simulink model "WaterRunner_closed"  (Simulink 8.0)
settings: Solver=ode15s  StartTime=0.0  StopTime=10  FixedStep=1e-3  RelTol=1e-3
values from neighbouring files (symbols this model uses):
  Amp = leg_length    (= 0.0428)    [SimParam.m]    (also in simParams_closed.m = 0.0249)
  b_water = 0.5*C_d*S1*density    (= 0.405708731037)    [SimParam.m]    (also in simParams_closed.m)
  D = 2*pi    (= 6.28318530718)    [DF_param.m]
  Filter_Coef = 1000    [SimParam.m]    (also in simParams_closed.m)
  frame_inertia = diag([Ix,Iy,Iz])    [SimParam.m]    (also in matlab.mat = [8.0125e-05  0  0; 0  0.000390625  0; 0  0  0.0003145]; simParams.m; simParams_closed.m; speed_cg.mat = [8.0125e-05  0  0; 0  0.000390625  0; 0  0  0.0003145])
  frame_mass = 0.06    [matlab.mat]    (also in simParam.m = 0.03; simParams.m; simParams_closed.m = 0.1; speed_cg.mat)
  Fratio = 1/16    (= 0.0625)    [SimParam.m]    (also in simParams_closed.m)
  g = 9.81    [SimParam.m]    (also in linear_search_df.m; simParams_closed.m)
  k_water = C_d*S1*density*g    (= 7.96000530294)    [SimParam.m]    (also in simParams_closed.m)
  L2_inertia = [1.05087286587e-08  0  0; 0  0  0; 0  0  1.05087286587e-08]    [matlab.mat]    (also in simParams.m = diag([I 0 I]); simParams_closed.m = diag([I 0 I]); speed_cg.mat)
  L2_mass = 0.0002653496    [matlab.mat]    (also in simParams.m; simParams_closed.m; speed_cg.mat)
  L3_inertia = [4.24507620885e-07  0  0; 0  0  0; 0  0  4.24507620885e-07]    [matlab.mat]    (also in simParams.m = diag([I 0 I]); simParams_closed.m = diag([I 0 I]); speed_cg.mat)
  L3_mass = 0.0009104656    [matlab.mat]    (also in simParams.m; simParams_closed.m; speed_cg.mat)
  L4_inertia = [1.03972444992e-07  0  0; 0  0  0; 0  0  1.03972444992e-07]    [matlab.mat]    (also in simParams.m = diag([I 0 I]); simParams_closed.m = diag([I 0 I]); speed_cg.mat)
  L4_mass = 0.0005696496    [matlab.mat]    (also in simParams.m; simParams_closed.m; speed_cg.mat)
  leg_length = 0.0428    [SimParam.m]    (also in simParams_closed.m = 0.0249)
  Lx = frame_width/2*[1 1 -1 -1]'    [SimParam.m]    (also in simParams_closed.m)
  Lxmat = frame_width/2*[1 0 0 0 ; 0 1 0 0 ; 0 0 -1 0 ; 0 0 0 -1]    [SimParam.m]    (also in simParams_closed.m)
  Lz = frame_length/2*[1 -1 -1 1]'    [SimParam.m]    (also in simParams_closed.m)
  Lzmat = frame_length/2*[1 0 0 0 ; 0 -1 0 0 ; 0 0 -1 0 ; 0 0 0 1]    [SimParam.m]    (also in simParams_closed.m)
  mass = 0.1    [SimParam.m]    (also in simParams_closed.m = 0.1581990592)
  mass_matrix = [mass 0 0; 0 Ix 0 ; 0 0 Iz]    [SimParam.m]    (also in simParams_closed.m)
  omega_0 = freq*ones(8,1)    [SimParam.m]    (also in simParams_closed.m)
  water_level = 0    [matlab.mat]    (also in simParam.m; simParams.m; simParams_closed.m; speed_cg.mat)
undefined symbols (not defined in the file): cw_FL_HL, cw_FR_FL, cw_FR_HR, cw_HR_HL, FL_HL_lag, FR_FL_lag, FR_HR_lag, freq, HR_HL_lag, initRobHeight, K_d, K_i, K_p, y_0
libraries: mblibv1 x17, WaterRunner_lib x14, dspstat3 x4, simulink x1, dspinverses x1
settings Model: Creator=fumiyaiida  LastModifiedBy=nitisht  SimulationMode=accelerator
settings SolverCC: ZeroCrossControl=DisableAll
settings DataIOCC: SignalLoggingSaveFormat=ModelDataLogs
settings OptimizationCC: InlineInvariantSignals=on  InitFltsAndDblsToZero=on  EfficientMapNaN2IntZero=off  SimCompilerOptimization=On
settings DebuggingCC: SaveWithParameterizedLinksMsg=none  SignalResolutionControl=TryResolveAllWithWarning  SolverPrmCheckMsg=none  MultiTaskDSMMsg=warning  MultiTaskCondExecSysMsg=none  FcnCallInpInsideContextMsg=UseLocalSettings  StrictBusMsg=None
settings HardwareCC: ProdBitPerLong=64  ProdBitPerPointer=64  ProdIntDivRoundTo=Zero  ProdEndianess=LittleEndian  ProdWordSize=64  ProdHWDeviceType=Intel->x86-64  TargetBitPerLong=64  TargetBitPerPointer=64  TargetIntDivRoundTo=Zero  TargetEndianess=LittleEndian  TargetWordSize=64  TargetHWDeviceType=MATLAB Host  ProdEqTarget=off
settings RTWCC: RTWCompilerOptimization=On
settings CodeAppCC: MaxIdLength=128
settings GRTTargetCC: CombineOutputUpdateFcns=off  GRTInterface=on
settings SimMechanicsCC: WarnOnSingularInitialAssembly=on  VisDuringSimulation=on  VisSampleTime=0.001  AnimationDelay=1  LastVizWinPosition=[1323 2 597 976]  CamPosition=[-7.43826;3.54067;9.27536;]  CamTarget=[0.848137;-0.562095;-0.541519;]  CamUpVector=[0.217493;0.952228;-0.21438;]  CamHeight=2.55  VisBackgroundColor=[0.9;0.9;0.95;]  DefaultBodyColor=[1;0;0;]
settings ConfigurationSet: Description=SimMechanics 2G

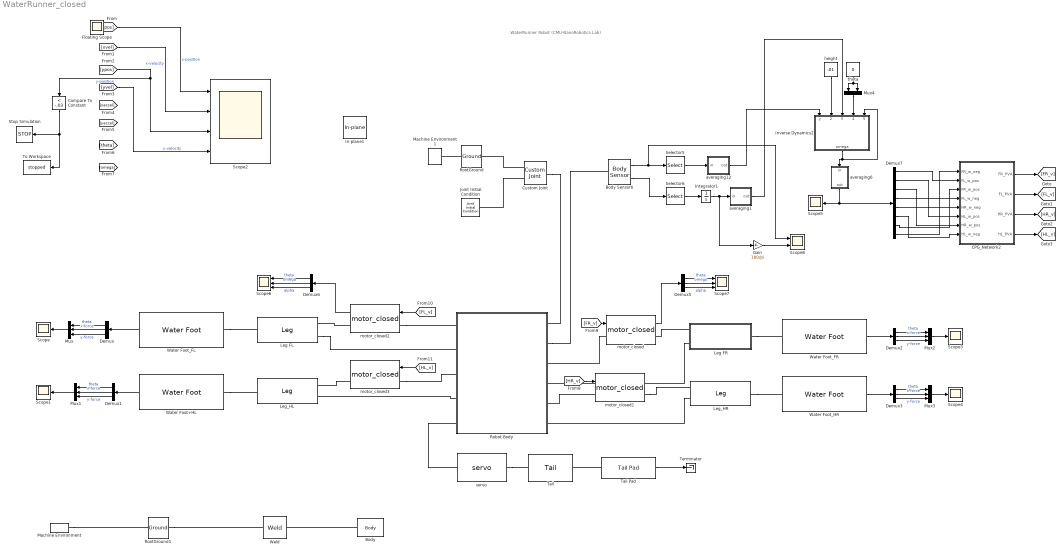
== system WaterRunner_closed ==
  note: WaterRunner Robot
      | (CMU-NanoRobotics Lab)
  Body : mblibv1/Bodies/Body  LConnTagsString=CG  UpdateFromCAD=off  DialogClass=MechanicalBodyBlock  Mass=1  MassUnits=kg  InertiaUnits=kg*m^2  Inertia=eye(3)  Shape=Cylinder  ShapeDims=[1 1]  ShapeUnits=m  ShapeUse=false  Density=1  DensityUnits=kg/m^3  DensityUse=false  GraphicsMode=CONVHULL  BodyColorSelMode=COLORPALETTE  BodyColor=[0.83137 0.81569 0.78431]  AttachedToCS=CG  CG=Left$CG$[0 0 0]$WORLD$WORLD$m$[0 0 0]$Euler X-Y-Z$deg$WORLD$true$none  WorkingFrames=Left$CS1$[-0.5 water_level -0.2 ]$CG$CG$m$[0 0 0]$Euler X-Y-Z$deg$WORLD$false$none#Left$CS2$[-0.5 water_level 0.2 ]$CG$CG$m$[0 0 0]$Euler X-Y-Z$deg$WORLD$false$none#Left$CS3$[4 water_level -0.2 ]$CG$CG$m$[0 0 0]$Euler X-Y-Z$deg$WORLD$false$none#Left$CS4$[4 water_level 0.2 ]$CG$CG$m$[0 0 0]$Euler X-Y-Z$deg$WORLD$false$none  CGPos=[0 0 0]  CGRot=[0 0 0]  CS0Pos=[]  CS0Rot=[]  CS1Pos=[-0.5 water_level -0.2 ]  CS1Rot=[0 0 0]  CS2Pos=[-0.5 water_level 0.2 ]  CS2Rot=[0 0 0]  CS3Pos=[4 water_level -0.2 ]  CS3Rot=[0 0 0]  CS4Pos=[4 water_level 0.2 ]  CS4Rot=[0 0 0]  CS5Pos=[]  CS5Rot=[]  CS6Pos=[]  CS6Rot=[]  CS7Pos=[]  CS7Rot=[]  CS8Pos=[]  CS8Rot=[]  CS9Pos=[]  CS9Rot=[]  CS10Pos=[]  CS10Rot=[]  CS11Pos=[]  CS11Rot=[]  CS12Pos=[]  CS12Rot=[]  CS13Pos=[]  CS13Rot=[]  CS14Pos=[]  CS14Rot=[]  CS15Pos=[]  CS15Rot=[]  CS16Pos=[]  CS16Rot=[]  CS17Pos=[]  CS17Rot=[]  CS18Pos=[]  CS18Rot=[]  CS19Pos=[]  CS19Rot=[]  CS20Pos=[]  CS20Rot=[]
  Body Sensor6 : mblibv1/Sensors &  Actuators/Body Sensor  UpdateFromCAD=off  PhysicalDomain=Mechanical  PortType=blob  Muxed=off  Pose=off  Angle=on  AngleUnits=deg  ArcVelocity=on  ArcVelocityUnits=rad/s  ArcAcceleration=off  ArcAccelerationUnits=deg/s^2  CoordPosition=on  CoordPositionUnits=m  Velocity=off  VelocityUnits=m/s  Acceleration=off  AccelerationUnits=m/s^2  Quaternion=on  QuaternionDT=off  QuaternionDDT=off  QuaternionUnits=off  OutputVector=[1]  ActiveIO=on  Width=6  DialogClass=MechanicalSensorBlock  ReferenceFrame=Absolute (World)
  CPG_Network2 : Subsystem
  Compare To Constant : simulink/Logic and Bit Operations/Compare To Constant  relop=<  const=-.03  OutDataTypeStr=boolean
  Custom Joint : mblibv1/Joints/Custom Joint  LConnTagsString=__newl0|SA1  RConnTagsString=__newr0  UpdateFromCAD=off  NumSAPorts=1  CutJoint=off  MarkAsCut=off  Primitives=prismatic  PrimitiveProps=P1$World$[0 1 0]$Prismatic#P2$World$[1 0 0]$Prismatic#R1$World$[1 0 0]$Revolute#R2$World$[0 0 1]$Revolute  DialogClass=JointBlock  R1Axis=[1 0 0]  R2Axis=[0 0 1]  R3Axis=[]  P1Axis=[0 1 0]  P2Axis=[1 0 0]  P3Axis=[]  SAxis=[]
  Demux{,1..3,5..6} (6 alike) : Demux  Outputs=3
  Demux7 : Demux  Outputs=8
  Gain : Gain  Gain=180/pi
  In-plane1 : mblibv1/Joints/In-plane  LConnTagsString=__newl0|SA1|SA2  RConnTagsString=__newr0|SA1|SA2  UpdateFromCAD=off  NumSAPorts=4  CutJoint=off  MarkAsCut=off  Primitives=prismatic  PrimitiveProps=P1$World$[1 0 0]$prismatic#P2$World$[0 1 0]$prismatic  DialogClass=JointBlock  P1Axis=[1 0 0]  P2Axis=[0 1 0]
  Integrator1 : Integrator
  Inverse Dynamics2 : Subsystem
  Joint Initial Condition : mblibv1/Sensors &  Actuators/Joint Initial Condition  UpdateFromCAD=off  LeftPortType=blob  RightPortType=blob  PhysicalDomain=mechanical  DialogClass=InitialConditionBlock  InitialConditions=P1$true$0$m$deg$0$m/s$deg/s#P2$false$initRobHeight$m$deg$0$m/s$deg/s#P3$false$0$m$deg$0$m/s$deg/s#R1$false$0$m$rad$0$m/s$rad/s#R2$false$0$m$deg$0$m/s$deg/s#R3$false$0$m$deg$0$m/s$deg/s#S$false$0$m$deg$0$m/s$deg/s  P1PIC=0  P1VIC=0  P2PIC=0  P2VIC=0  P3PIC=0  P3VIC=0  R1PIC=0  R1VIC=0  R2PIC=0  R2VIC=0  R3PIC=0  R3VIC=0  SPIC=0  SVIC=0
  Leg FL : WaterRunner_lib/Leg
  Leg FR : Subsystem  AncestorBlock=WaterRunner_lib/Leg
      mask help: mask for leg
  Leg_HL : WaterRunner_lib/Leg
  Leg_HR : WaterRunner_lib/Leg
  Machine Environment : mblibv1/Bodies/Machine Environment  PortType=env  PhysicalDomain=Mechanical  DialogTemplateClass=MECH.MachineEnvironment  SyncWhenCopied=off  Gravity=[0 -9.81 0]  GravityUnits=m/s^2  GravityAsSignal=off  Dimensionality=Auto-detect  AnalysisType=Forward dynamics  LinearAssemblyTolerance=1e-3  LinearAssemblyToleranceUnits=m  AngularAssemblyTolerance=1e-3  AngularAssemblyToleranceUnits=rad  ConstraintSolverType=Stabilizing  ConstraintRelTolerance=1e-4  ConstraintAbsTolerance=1e-4  UseRobustSingularityHandling=off  RedundancyAnalysisToleranceType=Automatically select tolerance  RedundancyAnalysisTolerance=1e-14  StatePerturbationType=Fixed  PerturbationSize=1e-5  VisualizeMachine=on  BodyVisualizationType=Use model default body geometries  BodyColorSelMode=Use model default  DefaultBodyColor=[1 0 0]
  Machine Environment1 : mblibv1/Bodies/Machine Environment  PortType=env  PhysicalDomain=Mechanical  DialogTemplateClass=MECH.MachineEnvironment  SyncWhenCopied=off  Gravity=[0 -9.81 0]  GravityUnits=m/s^2  GravityAsSignal=off  Dimensionality=Auto-detect  AnalysisType=Forward dynamics  LinearAssemblyTolerance=1e-3  LinearAssemblyToleranceUnits=m  AngularAssemblyTolerance=1e-3  AngularAssemblyToleranceUnits=rad  ConstraintSolverType=Stabilizing  ConstraintRelTolerance=1e-4  ConstraintAbsTolerance=1e-4  UseRobustSingularityHandling=off  RedundancyAnalysisToleranceType=Automatically select tolerance  RedundancyAnalysisTolerance=1e-14  StatePerturbationType=Fixed  PerturbationSize=1e-5  VisualizeMachine=on  BodyVisualizationType=Use model default body geometries  BodyColorSelMode=Use model default  DefaultBodyColor=[1 0 0]
  Mux{,1..3} (4 alike) : Mux  Inputs=3
  Mux4 : Mux  Inputs=2
  Robot Body : Subsystem  AncestorBlock=WaterRunner_lib/Robot Body  mask{initRobHeight=initRobHeight}
      mask prompts: initRobHeight "height"
  RootGround : mblibv1/Bodies/Ground  UpdateFromCAD=on  LeftPortType=env  RightPortType=workingframe  PhysicalDomain=Mechanical  DialogClass=GroundBlock  CoordPosition=[0 0 0]  CoordPositionUnits=m  StateVectorMgrId=-1  MachineId=[0 0]  ShowEnvPort=on
  RootGround1 : mblibv1/Bodies/Ground  UpdateFromCAD=on  LeftPortType=env  RightPortType=workingframe  PhysicalDomain=Mechanical  DialogClass=GroundBlock  CoordPosition=[0 0 0]  CoordPositionUnits=m  StateVectorMgrId=-1  MachineId=[0 0]  ShowEnvPort=on
  Scope{,1,3..5} (5 alike) : Scope
      Scope settings: ShowLegends=on  TimeRange=2  YMin=-2.5  YMax=2  SaveName=FootForce_FL
      Scope1 settings: ShowLegends=on  TimeRange=2  YMin=-2.5  YMax=2  SaveName=FootForce_HL
      Scope3 settings: ShowLegends=on  TimeRange=2  YMin=-2.5  YMax=2  SaveName=FootForce_FR
      Scope4 settings: ShowLegends=on  TimeRange=2  YMin=-2.5  YMax=2  SaveName=FootForce_HR
      Scope5 settings: TimeRange=30  YMin=15  YMax=125  SaveName=command_omega
  Scope2 : Scope  NumInputPorts=4
      settings: ShowLegends=on  TimeRange=10  YMin=-0.25~0~-0.005~-0.3  YMax=2~2.5~0.035~0.4  SaveName=position
  Scope6 : Scope  NumInputPorts=3
      settings: TimeRange=2  YMin=-20~-90~-50000  YMax=-2.5~0~30000  SaveName=MotorMotion1
  Scope7 : Scope  NumInputPorts=3
      settings: TimeRange=2  YMin=-17.5~-90~-70000  YMax=0~0~30000  SaveName=MotorMotion
  Scope8 : Scope  NumInputPorts=2
      settings: TimeRange=30  YMin=0.0015~-1.25  YMax=0.012~1.5  SaveName=ball_position
  Selector5 : Selector  InputPortWidth=3  IndexOptions=Index vector (dialog)  Indices=[2]  OutputSizes=1
  Selector6 : Selector  InputPortWidth=3  IndexOptions=Index vector (dialog)  Indices=[1 3]  OutputSizes=1
  Stop Simulation : Stop
  Tail : WaterRunner_lib/Tail
  Tail Pad : WaterRunner_lib/Tail Pad
  Terminator : Terminator
  To Workspace : ToWorkspace  VariableName=stopped  SampleTime=-1  SaveFormat=Timeseries
  Water Foot+HL : WaterRunner_lib/Water Foot
  Water Foot_FL : WaterRunner_lib/Water Foot
  Water Foot_FR : WaterRunner_lib/Water Foot
  Water Foot_HR : WaterRunner_lib/Water Foot
  Weld : mblibv1/Joints/Weld  LConnTagsString=__newl0  RConnTagsString=__newr0  UpdateFromCAD=off  NumSAPorts=0  CutJoint=off  MarkAsCut=off  Primitives=weld  PrimitiveProps=W$WORLD$[0 0 0]$weld  DialogClass=JointBlock  WAxis=[0 0 0]
  averaging1 : Subsystem  mask{T_win=2*pi/freq*4, x_init=[0, 0]}
      mask prompts: T_win "window (s)"; x_init "Initial condition"
  averaging12 : Subsystem  mask{T_win=2*pi/freq*4, x_init=y_0}
      mask prompts: T_win "window (s)"; x_init "Initial condition"
  averaging6 : Subsystem  mask{T_win=2*pi/freq, x_init=omega_0}
      mask prompts: T_win "window (s)"; x_init "Initial condition"
  height : Constant  Value=.01
  motor_closed : WaterRunner_lib/motor_closed  ic_angle=pi
  motor_closed1 : WaterRunner_lib/motor_closed  ic_angle=0
  motor_closed2 : WaterRunner_lib/motor_closed  ic_angle=0
  motor_closed3 : WaterRunner_lib/motor_closed  ic_angle=pi
  servo : WaterRunner_lib/servo  tail_angle=tail_angle  VariableName=work_tail
  theta : Constant  Value=0
  Floating Scope : Scope
      settings: Floating=on
  wires:
  Water Foot_FL/1 -> Demux/1
  Demux/1 -> Mux/1  "theta"
  Demux/2 -> Mux/2  "x-force"
  Demux/3 -> Mux/3  "y-force"
  Mux/1 -> Scope/1
  [ypos] -> Compare To Constant/1, Scope2/3  "y-position"
  Water Foot+HL/1 -> Demux1/1
  Demux1/1 -> Mux1/1  "theta"
  Demux1/2 -> Mux1/2  "x-force"
  Demux1/3 -> Mux1/3  "y-force"
  Mux1/1 -> Scope1/1
  Mux2/1 -> Scope3/1
  Demux2/3 -> Mux2/3  "y-force"
  Demux2/2 -> Mux2/2  "x-force"
  Demux2/1 -> Mux2/1  "theta"
  Water Foot_FR/1 -> Demux2/1
  Mux3/1 -> Scope4/1
  Demux3/3 -> Mux3/3  "y-force"
  Demux3/2 -> Mux3/2  "x-force"
  Demux3/1 -> Mux3/1  "theta"
  Water Foot_HR/1 -> Demux3/1
  Compare To Constant/1 -> To Workspace/1, Stop Simulation/1
  Demux5/3 -> Scope7/3  "alpha"
  Demux5/2 -> Scope7/2  "omega"
  Demux5/1 -> Scope7/1  "theta"
  motor_closed/1 -> Demux5/1
  Demux6/3 -> Scope6/3  "alpha"
  Demux6/2 -> Scope6/2  "omega"
  Demux6/1 -> Scope6/1  "theta"
  motor_closed2/1 -> Demux6/1
  Tail Pad/1 -> Terminator/1
  [xpos] -> Scope2/1  "x-position"
  [xvel] -> Scope2/2  "x-velocity"
  [yvel] -> Scope2/4  "y-velocity"
  CPG_Network2/1(FR_PVA) -> [FR_v]
  CPG_Network2/2(FL_PVA) -> [FL_v]
  CPG_Network2/3(HR_PVA) -> [HR_v]
  CPG_Network2/4(HL_PVA) -> [HL_v]
  [FR_v] -> motor_closed/1
  [HR_v] -> motor_closed1/1
  [FL_v] -> motor_closed2/1
  [HL_v] -> motor_closed3/1
  Inverse Dynamics2/1(omega) -> averaging6/1(in), Inverse Dynamics2/5(omega_last)
  Selector6/1 -> Integrator1/1
  Body Sensor6/2 -> Selector6/1
  Selector5/1 -> averaging12/1(in)
  Integrator1/1 -> Gain/1, averaging1/1(in)
  Gain/1 -> Scope8/2
  Body Sensor6/1 -> Scope8/1, Selector5/1
  height/1 -> Inverse Dynamics2/2(y_des)
  Mux4/1 -> Inverse Dynamics2/4(angle_des)
  theta/1 -> Mux4/1, Mux4/2
  averaging12/1(out) -> Inverse Dynamics2/1(y)
  averaging1/1(out) -> Inverse Dynamics2/3(angle)
  averaging6/1(out) -> Demux7/1, Scope5/1
  Demux7/8 -> CPG_Network2/1(FR_w_neg)
  Demux7/4 -> CPG_Network2/3(FR_w_pos)
  Demux7/1 -> CPG_Network2/2(FL_w_pos)
  Demux7/2 -> CPG_Network2/6(HL_w_pos)
  Demux7/3 -> CPG_Network2/7(HR_w_pos)
  Demux7/5 -> CPG_Network2/4(FL_w_neg)
  Demux7/6 -> CPG_Network2/8(HL_w_neg)
  Demux7/7 -> CPG_Network2/5(HR_w_neg)
  connections:
  RootGround1/RConn1 -- Weld/LConn1
  Body/LConn1 -- Weld/RConn1
  motor_closed/LConn1 -- Robot Body/RConn3
  Leg FR/LConn2 -- Robot Body/RConn4
  motor_closed/RConn1 -- Leg FR/LConn1
  motor_closed1/LConn1 -- Robot Body/RConn5
  motor_closed1/RConn1 -- Leg_HR/LConn1
  Leg_HR/LConn2 -- Robot Body/RConn6
  Water Foot+HL/LConn1 -- Leg_HL/RConn1
  Water Foot_FL/LConn1 -- Leg FL/RConn1
  Robot Body/LConn4 -- Leg_HL/LConn2
  Leg FR/RConn1 -- Water Foot_FR/LConn1
  Leg_HR/RConn1 -- Water Foot_HR/LConn1
  motor_closed2/LConn1 -- Robot Body/LConn1
  motor_closed3/RConn1 -- Leg_HL/LConn1
  motor_closed3/LConn1 -- Robot Body/LConn3
  Leg FL/LConn2 -- Robot Body/LConn2
  Machine Environment/RConn1 -- RootGround1/LConn1
  motor_closed2/RConn1 -- Leg FL/LConn1
  Robot Body/LConn5 -- servo/LConn1
  servo/RConn1 -- Tail/LConn1
  Tail Pad/LConn1 -- Tail/RConn1
  Custom Joint/LConn1 -- RootGround/RConn1
  Custom Joint/LConn2 -- Joint Initial Condition/RConn1
  RootGround/LConn1 -- Machine Environment1/RConn1
  Robot Body/RConn2 -- Body Sensor6/LConn1
  Custom Joint/RConn1 -- Robot Body/RConn1

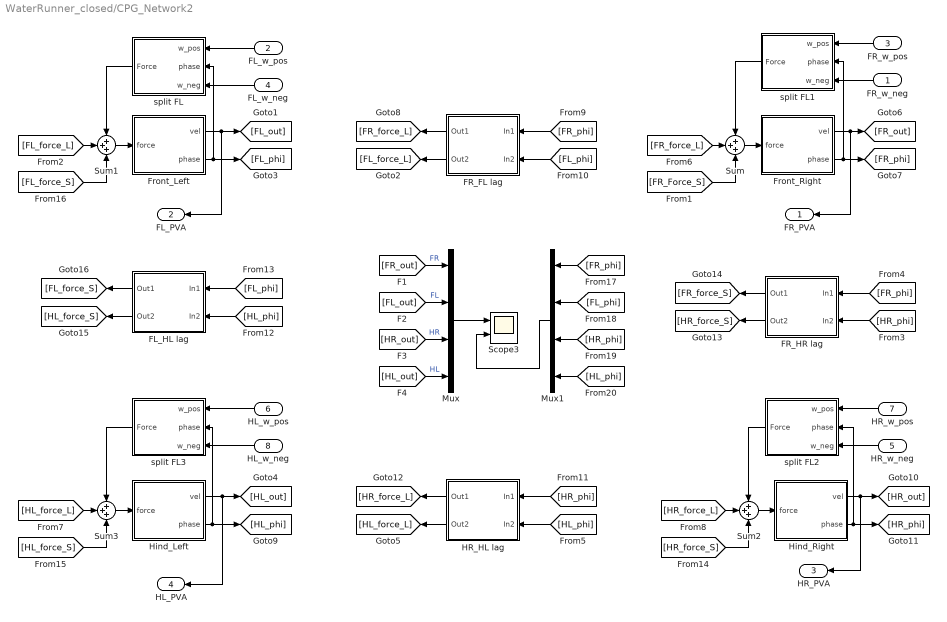
== system WaterRunner_closed/CPG_Network2 ==
  FR_w_neg : Inport
  FL_w_pos : Inport  Port=2
  FR_w_pos : Inport  Port=3
  FL_w_neg : Inport  Port=4
  HR_w_neg : Inport  Port=5
  HL_w_pos : Inport  Port=6
  HR_w_pos : Inport  Port=7
  HL_w_neg : Inport  Port=8
  FL_HL lag : Subsystem  mask{d_phase=FL_HL_lag, coupling_weight=cw_FL_HL}
      mask prompts: d_phase "Phase Lag"; coupling_weight "Coupling Weight"
  FR_FL lag : Subsystem  mask{d_phase=FR_FL_lag, coupling_weight=cw_FR_FL}
      mask prompts: d_phase "Phase Lag"; coupling_weight "Coupling Weight"
  FR_HR lag : Subsystem  mask{d_phase=FR_HR_lag, coupling_weight=cw_FR_HR}
      mask prompts: d_phase "Phase Lag"; coupling_weight "Coupling Weight"
  Front_Left : Subsystem  mask{init_phi=0}
      mask prompts: init_phi "Initial Phase"
  Front_Right : Subsystem  mask{init_phi=pi}
      mask prompts: init_phi "Initial Phase"
  HR_HL lag : Subsystem  mask{d_phase=HR_HL_lag, coupling_weight=cw_HR_HL}
      mask prompts: d_phase "Phase Lag"; coupling_weight "Coupling Weight"
  Hind_Left : Subsystem  mask{init_phi=pi}
      mask prompts: init_phi "Initial Phase"
  Hind_Right : Subsystem  mask{init_phi=0}
      mask prompts: init_phi "Initial Phase"
  Mux : Mux
  Mux1 : Mux
  Scope3 : Scope  NumInputPorts=2
      settings: ShowLegends=on  TimeRange=5  YMin=22.11~0  YMax=22.34~6.5  SaveName=Output
  Sum{,1..3} (4 alike) : Sum  Inputs=+++
  split FL : Subsystem
  split FL1 : Subsystem
  split FL2 : Subsystem
  split FL3 : Subsystem
  FR_PVA : Outport
  FL_PVA : Outport  Port=2
  HR_PVA : Outport  Port=3
  HL_PVA : Outport  Port=4
  wires:
  Mux/1 -> Scope3/1
  Front_Left/2(phase) -> split FL/2(phase), [FL_phi]
  Front_Right/2(phase) -> split FL1/2(phase), [FR_phi]
  [FL_phi] -> FR_FL lag/2(In2)
  [FR_phi] -> FR_FL lag/1(In1)
  FR_FL lag/1(Out1) -> [FR_force_L]
  FR_FL lag/2(Out2) -> [FL_force_L]
  Front_Right/1(vel) -> FR_PVA/1, [FR_out]
  [FL_force_L] -> Sum1/2
  Sum1/1 -> Front_Left/1(force)
  Sum/1 -> Front_Right/1(force)
  [FR_force_L] -> Sum/2
  [FL_out] -> Mux/2  "FL"
  [FR_out] -> Mux/1  "FR"
  FR_w_pos/1 -> split FL1/1(w_pos)
  FR_w_neg/1 -> split FL1/3(w_neg)
  split FL1/1(Force) -> Sum/1
  FL_w_pos/1 -> split FL/1(w_pos)
  FL_w_neg/1 -> split FL/3(w_neg)
  Front_Left/1(vel) -> FL_PVA/1, [FL_out]
  split FL/1(Force) -> Sum1/1
  Hind_Left/2(phase) -> split FL3/2(phase), [HL_phi]
  Hind_Right/2(phase) -> [HR_phi], split FL2/2(phase)
  [HL_phi] -> HR_HL lag/2(In2)
  [HR_phi] -> HR_HL lag/1(In1)
  HR_HL lag/1(Out1) -> [HR_force_L]
  HR_HL lag/2(Out2) -> [HL_force_L]
  Hind_Right/1(vel) -> HR_PVA/1, [HR_out]
  [HL_force_L] -> Sum3/2
  Sum3/1 -> Hind_Left/1(force)
  Sum2/1 -> Hind_Right/1(force)
  [HR_force_L] -> Sum2/2
  HR_w_pos/1 -> split FL2/1(w_pos)
  HR_w_neg/1 -> split FL2/3(w_neg)
  split FL2/1(Force) -> Sum2/1
  HL_w_pos/1 -> split FL3/1(w_pos)
  HL_w_neg/1 -> split FL3/3(w_neg)
  Hind_Left/1(vel) -> HL_PVA/1, [HL_out]
  split FL3/1(Force) -> Sum3/1
  [HR_phi] -> FR_HR lag/2(In2)
  [FR_phi] -> FR_HR lag/1(In1)
  FR_HR lag/1(Out1) -> [FR_force_S]
  FR_HR lag/2(Out2) -> [HR_force_S]
  [HL_phi] -> FL_HL lag/2(In2)
  [FL_phi] -> FL_HL lag/1(In1)
  FL_HL lag/1(Out1) -> [FL_force_S]
  FL_HL lag/2(Out2) -> [HL_force_S]
  [HL_out] -> Mux/4  "HL"
  [HR_out] -> Mux/3  "HR"
  [FR_Force_S] -> Sum/3
  [HR_force_S] -> Sum2/3
  [HL_force_S] -> Sum3/3
  [FL_force_S] -> Sum1/3
  Mux1/1 -> Scope3/2
  [FR_phi] -> Mux1/1
  [FL_phi] -> Mux1/2
  [HR_phi] -> Mux1/3
  [HL_phi] -> Mux1/4

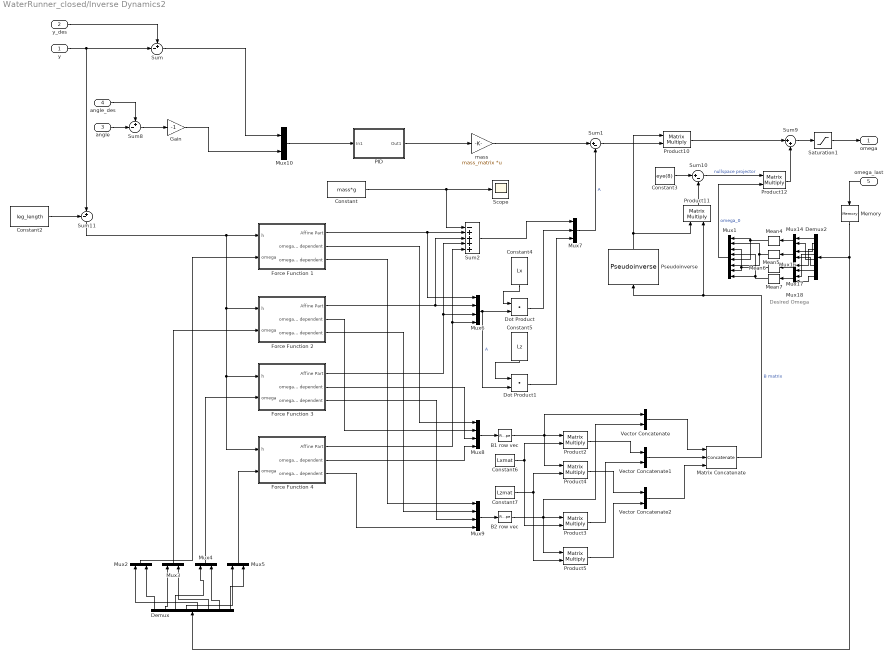
== system WaterRunner_closed/Inverse Dynamics2 ==
  note: Desired Omega
  y : Inport
  y_des : Inport  Port=2
  angle : Inport  Port=3
  angle_des : Inport  Port=4
  omega_last : Inport  Port=5
  B1 row vec : Reshape  OutputDimensionality=Row vector (2-D)  OutputDimensions=[1,2]
  B2 row vec : Reshape  OutputDimensionality=Row vector (2-D)  OutputDimensions=[1,2]
  Constant : Constant  Value=mass*g
  Constant2 : Constant  Value=leg_length
  Constant3 : Constant  Value=eye(8)
  Constant4 : Constant  Value=Lx
  Constant5 : Constant  Value=Lz
  Constant6 : Constant  Value=Lxmat
  Constant7 : Constant  Value=Lzmat
  Demux : Demux  Outputs=8
  Demux2 : Demux  Outputs=8
  Dot Product : DotProduct  InputSameDT=on  OutDataTypeStr=Inherit: Inherit via internal rule
  Dot Product1 : DotProduct  InputSameDT=on  OutDataTypeStr=Inherit: Inherit via internal rule
  Force Function 1 : Subsystem
  Force Function 2 : Subsystem
  Force Function 3 : Subsystem
  Force Function 4 : Subsystem
  Gain : Gain  Gain=-1
  Matrix Concatenate : Concatenate  NumInputs=3  Mode=Multidimensional array
  Mean{4..7} (4 alike) : dspstat3/Mean  run=off  reset_popup=None  InputProcessing=Columns as channels (frame based)  directionMode=Each column  dimension=1  treatSBRowAsCol=on  roiEnable=off  roiType=Rectangles  roiPortion=Entire ROI  roiOutput=Individual statistics for each ROI  roiFlag=off  outputDataTypeStr=Inherit: Same as accumulator  outputLastDataTypeStr=Inherit: Same as accumulator  outputMin=[]  outputMax=[]  roundingMode=Floor  overflowMode=off
  Memory : Memory  X0=omega_0
  Mux1 : Mux  Inputs=8
  Mux{2..5,10,14,16..18} (9 alike) : Mux  Inputs=2
  Mux6 : Mux
  Mux7 : Mux  Inputs=3
  Mux8 : Mux
  Mux9 : Mux
  PID : Subsystem  mask{P=K_p, I=K_i, D=K_d, N=Filter_Coef}
      mask prompts: P "Proportional Gain"; I "Integral Gain"; D "Derivative Gain"; N "Filter Coefficient"
  Product{2..5,10..12} (7 alike) : Product  Multiplication=Matrix(*)  RndMeth=Zero
  Pseudoinverse : dspinverses/Pseudoinverse  wanterr=off
  Saturation1 : Saturate  UpperLimit=120  LowerLimit=20
  Scope : Scope
      settings: YMin=0.972  YMax=0.9815
  Sum : Sum  Inputs=+-|
  Sum1 : Sum  Inputs=|+-
  Sum10 : Sum  Inputs=|+-
  Sum11 : Sum  Inputs=-+|
  Sum2 : Sum  Inputs=-++++
  Sum8 : Sum  Inputs=+-|
  Sum9 : Sum  Inputs=|++
  Vector Concatenate : Concatenate  ConcatenateDimension=2
  Vector Concatenate1 : Concatenate  ConcatenateDimension=2
  Vector Concatenate2 : Concatenate  ConcatenateDimension=2
  mass : Gain  Gain=mass_matrix  Multiplication=Matrix(K*u)
  omega : Outport
  wires:
  Memory/1 -> Demux2/1, Demux/1
  PID/1(Out1) -> mass/1
  y/1 -> Sum/2, Sum11/2
  Pseudoinverse/1 -> Product11/1, Product10/1
  Sum1/1 -> Product10/2
  Product10/1 -> Sum9/1
  Product11/1 -> Sum10/2
  Constant3/1 -> Sum10/1
  Sum10/1 -> Product12/1  "nullspace projector"
  Product12/1 -> Sum9/2
  Mux1/1 -> Product12/2  "omega_0"
  Force Function 1/1(Affine Part) -> Mux6/1, Sum2/2
  Force Function 2/1(Affine Part) -> Sum2/3, Mux6/2
  Force Function 3/1(Affine Part) -> Mux6/3, Sum2/4
  Force Function 4/1(Affine Part) -> Mux6/4, Sum2/5
  Mux6/1 -> Dot Product/2, Dot Product1/2  "A"
  Constant4/1 -> Dot Product/1
  Constant5/1 -> Dot Product1/1
  Sum2/1 -> Mux7/1
  Dot Product/1 -> Mux7/2
  Dot Product1/1 -> Mux7/3
  Mux7/1 -> Sum1/2  "A"
  Force Function 1/2(omega1 dependent) -> Mux8/1
  Force Function 2/2(omega1 dependent) -> Mux8/2
  Force Function 3/2(omega1 dependent) -> Mux8/3
  Force Function 1/3(omega2 dependent) -> Mux9/1
  Force Function 2/3(omega2 dependent) -> Mux9/2
  Force Function 4/2(omega1 dependent) -> Mux8/4
  Force Function 3/3(omega2 dependent) -> Mux9/3
  Force Function 4/3(omega2 dependent) -> Mux9/4
  Mux8/1 -> B1 row vec/1
  Mux9/1 -> B2 row vec/1
  B1 row vec/1 -> Vector Concatenate/1, Product4/1, Product2/1
  B2 row vec/1 -> Vector Concatenate/2, Product5/1, Product3/1
  Constant6/1 -> Product3/2, Product2/2
  Constant7/1 -> Product4/2, Product5/2
  Product2/1 -> Vector Concatenate1/1
  Product3/1 -> Vector Concatenate1/2
  Product4/1 -> Vector Concatenate2/1
  Product5/1 -> Vector Concatenate2/2
  Vector Concatenate/1 -> Matrix Concatenate/1
  Vector Concatenate1/1 -> Matrix Concatenate/2
  Vector Concatenate2/1 -> Matrix Concatenate/3
  Matrix Concatenate/1 -> Product11/2, Pseudoinverse/1  "B matrix"
  y_des/1 -> Sum/1
  Sum9/1 -> Saturation1/1
  Saturation1/1 -> omega/1
  mass/1 -> Sum1/1
  Constant/1 -> Scope/1, Sum2/1
  angle_des/1 -> Sum8/1
  angle/1 -> Sum8/2
  Sum8/1 -> Gain/1
  Sum/1 -> Mux10/1
  Gain/1 -> Mux10/2
  Mux10/1 -> PID/1(In1)
  omega_last/1 -> Memory/1
  Demux2/1 -> Mux14/1
  Demux2/5 -> Mux14/2
  Mux14/1 -> Mean4/1
  Mux16/1 -> Mean5/1
  Demux2/2 -> Mux16/1
  Demux2/6 -> Mux16/2
  Mux17/1 -> Mean6/1
  Mux18/1 -> Mean7/1
  Demux2/3 -> Mux17/1
  Demux2/7 -> Mux17/2
  Demux2/4 -> Mux18/1
  Demux2/8 -> Mux18/2
  Mean4/1 -> Mux1/1, Mux1/5
  Mean5/1 -> Mux1/2, Mux1/6
  Mean6/1 -> Mux1/7, Mux1/3
  Mean7/1 -> Mux1/8, Mux1/4
  Mux2/1 -> Force Function 1/2(omega)
  Mux3/1 -> Force Function 2/2(omega)
  Mux4/1 -> Force Function 3/2(omega)
  Mux5/1 -> Force Function 4/2(omega)
  Demux/5 -> Mux2/1
  Demux/1 -> Mux2/2
  Demux/2 -> Mux3/1
  Demux/6 -> Mux3/2
  Demux/3 -> Mux4/1
  Demux/4 -> Mux5/1
  Demux/7 -> Mux4/2
  Demux/8 -> Mux5/2
  Constant2/1 -> Sum11/1
  Sum11/1 -> Force Function 4/1(h), Force Function 3/1(h), Force Function 2/1(h), Force Function 1/1(h)

== system WaterRunner_closed/Leg FR ==
  L2_segment : mblibv1/Bodies/Body  LConnTagsString=CS1  RConnTagsString=CS2  UpdateFromCAD=off  DialogClass=MechanicalBodyBlock  Mass=L2_mass  MassUnits=kg  InertiaUnits=kg*m^2  Inertia=L2_inertia  Shape=Cylinder  ShapeDims=[1 1]  ShapeUnits=m  ShapeUse=false  Density=1  DensityUnits=kg/m^3  DensityUse=false  GraphicsMode=CONVHULL  BodyColorSelMode=COLORPALETTE  BodyColor=[0 0 0]  AttachedToCS=CG  CG=Left$CG$L2_CG$CS1$CS1$m$[0 0 0]$Euler X-Y-Z$deg$WORLD$false$none  WorkingFrames=Left$CS1$L2_CS1$Adjoining$Adjoining$m$[0 0 0]$Euler X-Y-Z$deg$WORLD$true$none#Right$CS2$L2_CS2$CS1$CS1$m$[0 0 0]$Euler X-Y-Z$deg$WORLD$true$none  CGPos=L2_CG  CGRot=[0 0 0]  CS0Pos=[]  CS0Rot=[]  CS1Pos=L2_CS1  CS1Rot=[0 0 0]  CS2Pos=L2_CS2  CS2Rot=[0 0 0]  CS3Pos=[]  CS3Rot=[]  CS4Pos=[]  CS4Rot=[]  CS5Pos=[]  CS5Rot=[]  CS6Pos=[]  CS6Rot=[]  CS7Pos=[]  CS7Rot=[]  CS8Pos=[]  CS8Rot=[]  CS9Pos=[]  CS9Rot=[]  CS10Pos=[]  CS10Rot=[]  CS11Pos=[]  CS11Rot=[]  CS12Pos=[]  CS12Rot=[]  CS13Pos=[]  CS13Rot=[]  CS14Pos=[]  CS14Rot=[]  CS15Pos=[]  CS15Rot=[]  CS16Pos=[]  CS16Rot=[]  CS17Pos=[]  CS17Rot=[]  CS18Pos=[]  CS18Rot=[]  CS19Pos=[]  CS19Rot=[]  CS20Pos=[]  CS20Rot=[]
  L3_segment : mblibv1/Bodies/Body  LConnTagsString=CS1  RConnTagsString=CS2|CS3  UpdateFromCAD=off  DialogClass=MechanicalBodyBlock  Mass=L3_mass  MassUnits=kg  InertiaUnits=kg*m^2  Inertia=L3_inertia  Shape=Cylinder  ShapeDims=[1 1]  ShapeUnits=m  ShapeUse=false  Density=1  DensityUnits=kg/m^3  DensityUse=false  GraphicsMode=CONVHULL  BodyColorSelMode=COLORPALETTE  BodyColor=[0 0 0]  AttachedToCS=CG  CG=Left$CG$L3_CG$CS1$CS1$m$[0 0 0]$Euler X-Y-Z$rad$CS1$false$none  WorkingFrames=Left$CS1$L3_CS1$Adjoining$Adjoining$m$L3_ori$Euler X-Y-Z$rad$Adjoining$true$none#Right$CS2$L3_CS2$CS1$CS1$m$[0 0 0]$Euler X-Y-Z$rad$CS1$true$none#Right$CS3$L3_CS3$CS1$CS1$m$[0 0 0]$Euler X-Y-Z$rad$CS1$true$none  CGPos=L3_CG  CGRot=[0 0 0]  CS0Pos=[]  CS0Rot=[]  CS1Pos=L3_CS1  CS1Rot=L3_ori  CS2Pos=L3_CS2  CS2Rot=[0 0 0]  CS3Pos=L3_CS3  CS3Rot=[0 0 0]  CS4Pos=[]  CS4Rot=[]  CS5Pos=[]  CS5Rot=[]  CS6Pos=[]  CS6Rot=[]  CS7Pos=[]  CS7Rot=[]  CS8Pos=[]  CS8Rot=[]  CS9Pos=[]  CS9Rot=[]  CS10Pos=[]  CS10Rot=[]  CS11Pos=[]  CS11Rot=[]  CS12Pos=[]  CS12Rot=[]  CS13Pos=[]  CS13Rot=[]  CS14Pos=[]  CS14Rot=[]  CS15Pos=[]  CS15Rot=[]  CS16Pos=[]  CS16Rot=[]  CS17Pos=[]  CS17Rot=[]  CS18Pos=[]  CS18Rot=[]  CS19Pos=[]  CS19Rot=[]  CS20Pos=[]  CS20Rot=[]
  L4_segment : mblibv1/Bodies/Body  LConnTagsString=CS1  RConnTagsString=CS2  UpdateFromCAD=off  DialogClass=MechanicalBodyBlock  Mass=L4_mass  MassUnits=kg  InertiaUnits=kg*m^2  Inertia=L4_inertia  Shape=Cylinder  ShapeDims=[1 1]  ShapeUnits=m  ShapeUse=false  Density=1  DensityUnits=kg/m^3  DensityUse=false  GraphicsMode=CONVHULL  BodyColorSelMode=COLORPALETTE  BodyColor=[0 0 0]  AttachedToCS=CG  CG=Left$CG$L4_CG$CS1$CS1$m$[0 0 0]$Euler X-Y-Z$rad$CS1$false$none  WorkingFrames=Left$CS1$L4_CS1$Adjoining$Adjoining$m$L4_ori$Euler X-Y-Z$rad$Adjoining$true$none#Right$CS2$L4_CS2$CS1$CS1$m$[0 0 0]$Euler X-Y-Z$rad$CS1$true$none  CGPos=L4_CG  CGRot=[0 0 0]  CS0Pos=[]  CS0Rot=[]  CS1Pos=L4_CS1  CS1Rot=L4_ori  CS2Pos=L4_CS2  CS2Rot=[0 0 0]  CS3Pos=[]  CS3Rot=[]  CS4Pos=[]  CS4Rot=[]  CS5Pos=[]  CS5Rot=[]  CS6Pos=[]  CS6Rot=[]  CS7Pos=[]  CS7Rot=[]  CS8Pos=[]  CS8Rot=[]  CS9Pos=[]  CS9Rot=[]  CS10Pos=[]  CS10Rot=[]  CS11Pos=[]  CS11Rot=[]  CS12Pos=[]  CS12Rot=[]  CS13Pos=[]  CS13Rot=[]  CS14Pos=[]  CS14Rot=[]  CS15Pos=[]  CS15Rot=[]  CS16Pos=[]  CS16Rot=[]  CS17Pos=[]  CS17Rot=[]  CS18Pos=[]  CS18Rot=[]  CS19Pos=[]  CS19Rot=[]  CS20Pos=[]  CS20Rot=[]
  Revolute1 : mblibv1/Joints/Revolute  LConnTagsString=__newl0  RConnTagsString=__newr0  UpdateFromCAD=off  NumSAPorts=0  CutJoint=off  MarkAsCut=off  Primitives=prismatic  PrimitiveProps=R1$World$[0 0 1]$revolute  DialogClass=JointBlock  R1Axis=[0 0 1]
  Revolute2 : mblibv1/Joints/Revolute  LConnTagsString=__newl0  RConnTagsString=__newr0  UpdateFromCAD=off  NumSAPorts=0  CutJoint=on  MarkAsCut=off  Primitives=prismatic  PrimitiveProps=R1$World$[0 0 1]$revolute  DialogClass=JointBlock  R1Axis=[0 0 1]
  Revolute3 : mblibv1/Joints/Revolute  LConnTagsString=__newl0  RConnTagsString=__newr0  UpdateFromCAD=off  NumSAPorts=0  CutJoint=off  MarkAsCut=off  Primitives=prismatic  PrimitiveProps=R1$World$[0 0 1]$revolute  DialogClass=JointBlock  R1Axis=[0 0 1]
  motor : PMIOPort  Port=1  Side=Left
  end : PMIOPort  Port=2  Side=Right
  body : PMIOPort  Port=3  Side=Left
  connections:
  L2_segment/LConn1 -- motor/RConn1
  Revolute2/LConn1 -- L2_segment/RConn1
  L3_segment/LConn1 -- Revolute2/RConn1
  L3_segment/RConn1 -- Revolute3/RConn1
  Revolute1/RConn1 -- L4_segment/LConn1
  Revolute3/LConn1 -- L4_segment/RConn1
  body/RConn1 -- Revolute1/LConn1
  end/RConn1 -- L3_segment/RConn2

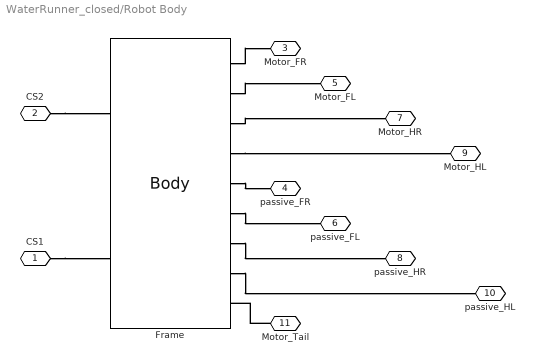
== system WaterRunner_closed/Robot Body ==
  Frame : mblibv1/Bodies/Body  LConnTagsString=CG|CS1  RConnTagsString=CS6|CS7|CS8|CS9|CS10|CS11|CS12|CS13|CS14  UpdateFromCAD=off  DialogClass=MechanicalBodyBlock  Mass=frame_mass  MassUnits=kg  InertiaUnits=kg*m^2  Inertia=frame_inertia  Shape=Cylinder  ShapeDims=[1 1]  ShapeUnits=m  ShapeUse=false  Density=1  DensityUnits=kg/m^3  DensityUse=false  GraphicsMode=CONVHULL  BodyColorSelMode=COLORPALETTE  BodyColor=[0 0 1]  AttachedToCS=CG  CG=Left$CG$frame_CG$WORLD$WORLD$m$[0 0 0]$Euler X-Y-Z$deg$WORLD$true$none  WorkingFrames=Left$CS1$frame_CA$World$World$m$[0 0 0]$Euler X-Y-Z$deg$WORLD$true$none#Right$CS2$frame_FR$World$World$m$[0 0 0]$Euler X-Y-Z$deg$WORLD$false$none#Right$CS4$frame_FL$World$World$m$[0 0 0]$Euler X-Y-Z$deg$WORLD$false$none#Right$CS3$frame_HR$World$World$m$[0 0 0]$Euler X-Y-Z$deg$WORLD$false$none#Right$CS5$frame_HL$WORLD$WORLD$m$[0 0 0]$Euler X-Y-Z$deg$WORLD$false$none#Right$CS6$frame_motor_FR$WORLD$WORLD$m$[0 0 0]$Euler X-Y-Z$deg$WORLD$true$none#Right$CS7$frame_motor_FL$WORLD$WORLD$m$[0 0 0]$Euler X-Y-Z$deg$WORLD$true$none#Right$CS8$frame_motor_HR$WORLD$WORLD$m$[0 0 0]$Euler X-Y-Z$deg$WORLD$true$none#Right$CS9$frame_motor_HL$WORLD$WORLD$m$[0 0 0]$Euler X-Y-Z$deg$WORLD$true$none#Right$CS10$frame_passive_FR$WORLD$WORLD$m$[0 0 0]$Euler X-Y-Z$deg$WORLD$true$none#Right$CS11$frame_passive_FL$WORLD$WORLD$m$[0 0 0]$Euler X-Y-Z$deg$WORLD$true$none#Right$CS12$frame_passive_HR$WORLD$WORLD$m$[0 0 0]$Euler X-Y-Z$deg$WORLD$true$none#Right$CS13$frame_passive_HL$WORLD$WORLD$m$[0 0 0]$Euler X-Y-Z$deg$WORLD$true$none#Right$CS14$frame_motor_Tail$WORLD$WORLD$m$[0 0 0]$Euler X-Y-Z$deg$WORLD$true$none  CGPos=frame_CG  CGRot=[0 0 0]  CS0Pos=[]  CS0Rot=[]  CS1Pos=frame_CA  CS1Rot=[0 0 0]  CS2Pos=frame_FR  CS2Rot=[0 0 0]  CS3Pos=frame_HR  CS3Rot=[0 0 0]  CS4Pos=frame_FL  CS4Rot=[0 0 0]  CS5Pos=frame_HL  CS5Rot=[0 0 0]  CS6Pos=frame_motor_FR  CS6Rot=[0 0 0]  CS7Pos=frame_motor_FL  CS7Rot=[0 0 0]  CS8Pos=frame_motor_HR  CS8Rot=[0 0 0]  CS9Pos=frame_motor_HL  CS9Rot=[0 0 0]  CS10Pos=frame_passive_FR  CS10Rot=[0 0 0]  CS11Pos=frame_passive_FL  CS11Rot=[0 0 0]  CS12Pos=frame_passive_HR  CS12Rot=[0 0 0]  CS13Pos=frame_passive_HL  CS13Rot=[0 0 0]  CS14Pos=frame_motor_Tail  CS14Rot=[0 0 0]  CS15Pos=[]  CS15Rot=[]  CS16Pos=[]  CS16Rot=[]  CS17Pos=[]  CS17Rot=[]  CS18Pos=[]  CS18Rot=[]  CS19Pos=[]  CS19Rot=[]  CS20Pos=[]  CS20Rot=[]
  CS1 : PMIOPort  Port=1  Side=Right
  CS2 : PMIOPort  Port=2  Side=Right
  Motor_FR : PMIOPort  Port=3  Side=Right
  passive_FR : PMIOPort  Port=4  Side=Right
  Motor_FL : PMIOPort  Port=5  Side=Left
  passive_FL : PMIOPort  Port=6  Side=Left
  Motor_HR : PMIOPort  Port=7  Side=Right
  passive_HR : PMIOPort  Port=8  Side=Right
  Motor_HL : PMIOPort  Port=9  Side=Left
  passive_HL : PMIOPort  Port=10  Side=Left
  Motor_Tail : PMIOPort  Port=11  Side=Left
  connections:
  Motor_Tail/RConn1 -- Frame/RConn9
  Frame/RConn8 -- passive_HL/RConn1
  Frame/RConn7 -- passive_HR/RConn1
  Frame/RConn6 -- passive_FL/RConn1
  Frame/RConn5 -- passive_FR/RConn1
  Frame/RConn4 -- Motor_HL/RConn1
  Frame/RConn3 -- Motor_HR/RConn1
  Frame/RConn2 -- Motor_FL/RConn1
  Frame/RConn1 -- Motor_FR/RConn1
  CS1/RConn1 -- Frame/LConn2
  CS2/RConn1 -- Frame/LConn1

== system WaterRunner_closed/averaging1 ==
  in : Inport
  Constant1 : Constant  Value=x_init
  Gain : Gain  Gain=1/T_win
  Integrator1 : Integrator
  Sum : Sum  Inputs=+-|
  Sum1 : Sum  Inputs=-+|
  Sum3 : Sum  Inputs=++|
  Transport Delay : TransportDelay  DelayTime=T_win
  out : Outport
  wires:
  in/1 -> Sum1/2
  Gain/1 -> Sum3/2
  Constant1/1 -> Sum3/1, Sum1/1
  Sum1/1 -> Integrator1/1
  Transport Delay/1 -> Sum/2
  Integrator1/1 -> Sum/1, Transport Delay/1
  Sum3/1 -> out/1
  Sum/1 -> Gain/1

== system WaterRunner_closed/averaging12 ==
  in : Inport
  Constant1 : Constant  Value=x_init
  Gain : Gain  Gain=1/T_win
  Integrator1 : Integrator
  Sum : Sum  Inputs=+-|
  Sum1 : Sum  Inputs=-+|
  Sum3 : Sum  Inputs=++|
  Transport Delay : TransportDelay  DelayTime=T_win
  out : Outport
  wires:
  in/1 -> Sum1/2
  Gain/1 -> Sum3/2
  Constant1/1 -> Sum3/1, Sum1/1
  Sum1/1 -> Integrator1/1
  Transport Delay/1 -> Sum/2
  Integrator1/1 -> Sum/1, Transport Delay/1
  Sum3/1 -> out/1
  Sum/1 -> Gain/1

== system WaterRunner_closed/averaging6 ==
  in : Inport
  Constant1 : Constant  Value=x_init
  Gain : Gain  Gain=1/T_win
  Integrator1 : Integrator
  Sum : Sum  Inputs=+-|
  Sum1 : Sum  Inputs=-+|
  Sum3 : Sum  Inputs=++|
  Transport Delay : TransportDelay  DelayTime=T_win
  out : Outport
  wires:
  in/1 -> Sum1/2
  Gain/1 -> Sum3/2
  Constant1/1 -> Sum3/1, Sum1/1
  Sum1/1 -> Integrator1/1
  Transport Delay/1 -> Sum/2
  Integrator1/1 -> Sum/1, Transport Delay/1
  Sum3/1 -> out/1
  Sum/1 -> Gain/1

== system WaterRunner_closed/CPG_Network2/FL_HL lag ==
  In1 : Inport
  In2 : Inport  Port=2
  Constant : Constant  Value=d_phase
  Gain : Gain  Gain=-1
  Sum : Sum  Inputs=--+
  sin : Fcn  Expr=coupling_weight*sin(u(1))
  Out1 : Outport
  Out2 : Outport  Port=2
  wires:
  Sum/1 -> sin/1
  sin/1 -> Gain/1, Out1/1
  Constant/1 -> Sum/2
  In1/1 -> Sum/1
  In2/1 -> Sum/3
  Gain/1 -> Out2/1

== system WaterRunner_closed/CPG_Network2/FR_FL lag ==
  In1 : Inport
  In2 : Inport  Port=2
  Constant : Constant  Value=d_phase
  Gain : Gain  Gain=-1
  Sum : Sum  Inputs=--+
  sin : Fcn  Expr=coupling_weight*sin(u(1))
  Out1 : Outport
  Out2 : Outport  Port=2
  wires:
  Sum/1 -> sin/1
  sin/1 -> Gain/1, Out1/1
  Constant/1 -> Sum/2
  In1/1 -> Sum/1
  In2/1 -> Sum/3
  Gain/1 -> Out2/1

== system WaterRunner_closed/CPG_Network2/FR_HR lag ==
  In1 : Inport
  In2 : Inport  Port=2
  Constant : Constant  Value=d_phase
  Gain : Gain  Gain=-1
  Sum : Sum  Inputs=--+
  sin : Fcn  Expr=coupling_weight*sin(u(1))
  Out1 : Outport
  Out2 : Outport  Port=2
  wires:
  Gain/1 -> Out2/1
  In2/1 -> Sum/3
  In1/1 -> Sum/1
  Constant/1 -> Sum/2
  sin/1 -> Out1/1, Gain/1
  Sum/1 -> sin/1

== system WaterRunner_closed/CPG_Network2/Front_Left ==
  force : Inport
  Integrator3 : Integrator  InitialCondition=init_phi + 0.001*rand
  Mod 2pi : Fcn  Expr=atan2(sin(u(1)-pi),cos(u(1)-pi))+pi
  vel : Outport
  phase : Outport  Port=2
  wires:
  force/1 -> vel/1, Integrator3/1
  Integrator3/1 -> Mod 2pi/1
  Mod 2pi/1 -> phase/1

== system WaterRunner_closed/CPG_Network2/Front_Right ==
  force : Inport
  Integrator3 : Integrator  InitialCondition=init_phi + 0.001*rand
  Mod 2pi : Fcn  Expr=atan2(sin(u(1)-pi),cos(u(1)-pi))+pi
  vel : Outport
  phase : Outport  Port=2
  wires:
  Mod 2pi/1 -> phase/1
  Integrator3/1 -> Mod 2pi/1
  force/1 -> Integrator3/1, vel/1

== system WaterRunner_closed/CPG_Network2/HR_HL lag ==
  In1 : Inport
  In2 : Inport  Port=2
  Constant : Constant  Value=d_phase
  Gain : Gain  Gain=-1
  Sum : Sum  Inputs=--+
  sin : Fcn  Expr=coupling_weight*sin(u(1))
  Out1 : Outport
  Out2 : Outport  Port=2
  wires:
  Gain/1 -> Out2/1
  In2/1 -> Sum/3
  In1/1 -> Sum/1
  Constant/1 -> Sum/2
  sin/1 -> Out1/1, Gain/1
  Sum/1 -> sin/1

== system WaterRunner_closed/CPG_Network2/Hind_Left ==
  force : Inport
  Integrator3 : Integrator  InitialCondition=init_phi + 0.001*rand
  Mod 2pi : Fcn  Expr=atan2(sin(u(1)-pi),cos(u(1)-pi))+pi
  vel : Outport
  phase : Outport  Port=2
  wires:
  force/1 -> vel/1, Integrator3/1
  Integrator3/1 -> Mod 2pi/1
  Mod 2pi/1 -> phase/1

== system WaterRunner_closed/CPG_Network2/Hind_Right ==
  force : Inport
  Integrator3 : Integrator  InitialCondition=init_phi + 0.001*rand
  Mod 2pi : Fcn  Expr=atan2(sin(u(1)-pi),cos(u(1)-pi))+pi
  vel : Outport
  phase : Outport  Port=2
  wires:
  force/1 -> vel/1, Integrator3/1
  Integrator3/1 -> Mod 2pi/1
  Mod 2pi/1 -> phase/1

== system WaterRunner_closed/CPG_Network2/split FL ==
  w_pos : Inport
  phase : Inport  Port=2
  w_neg : Inport  Port=3
  Product : Product  RndMeth=Zero
  Product1 : Product  RndMeth=Zero
  Sum2 : Sum  Inputs=|++
  enable : Subsystem
  Force : Outport
  wires:
  Product/1 -> Sum2/1
  w_pos/1 -> Product/1
  w_neg/1 -> Product1/1
  Product1/1 -> Sum2/2
  enable/1(pos) -> Product/2
  enable/2(neg) -> Product1/2
  Sum2/1 -> Force/1
  phase/1 -> enable/1(in)

== system WaterRunner_closed/CPG_Network2/split FL1 ==
  w_pos : Inport
  phase : Inport  Port=2
  w_neg : Inport  Port=3
  Product : Product  RndMeth=Zero
  Product1 : Product  RndMeth=Zero
  Sum2 : Sum  Inputs=|++
  enable : Subsystem
  Force : Outport
  wires:
  Product/1 -> Sum2/1
  w_pos/1 -> Product/1
  w_neg/1 -> Product1/1
  Product1/1 -> Sum2/2
  enable/1(pos) -> Product/2
  enable/2(neg) -> Product1/2
  Sum2/1 -> Force/1
  phase/1 -> enable/1(in)

== system WaterRunner_closed/CPG_Network2/split FL2 ==
  w_pos : Inport
  phase : Inport  Port=2
  w_neg : Inport  Port=3
  Product : Product  RndMeth=Zero
  Product1 : Product  RndMeth=Zero
  Sum2 : Sum  Inputs=|++
  enable : Subsystem
  Force : Outport
  wires:
  phase/1 -> enable/1(in)
  Sum2/1 -> Force/1
  enable/2(neg) -> Product1/2
  enable/1(pos) -> Product/2
  Product1/1 -> Sum2/2
  w_neg/1 -> Product1/1
  w_pos/1 -> Product/1
  Product/1 -> Sum2/1

== system WaterRunner_closed/CPG_Network2/split FL3 ==
  w_pos : Inport
  phase : Inport  Port=2
  w_neg : Inport  Port=3
  Product : Product  RndMeth=Zero
  Product1 : Product  RndMeth=Zero
  Sum2 : Sum  Inputs=|++
  enable : Subsystem
  Force : Outport
  wires:
  Product/1 -> Sum2/1
  w_pos/1 -> Product/1
  w_neg/1 -> Product1/1
  Product1/1 -> Sum2/2
  enable/1(pos) -> Product/2
  enable/2(neg) -> Product1/2
  Sum2/1 -> Force/1
  phase/1 -> enable/1(in)

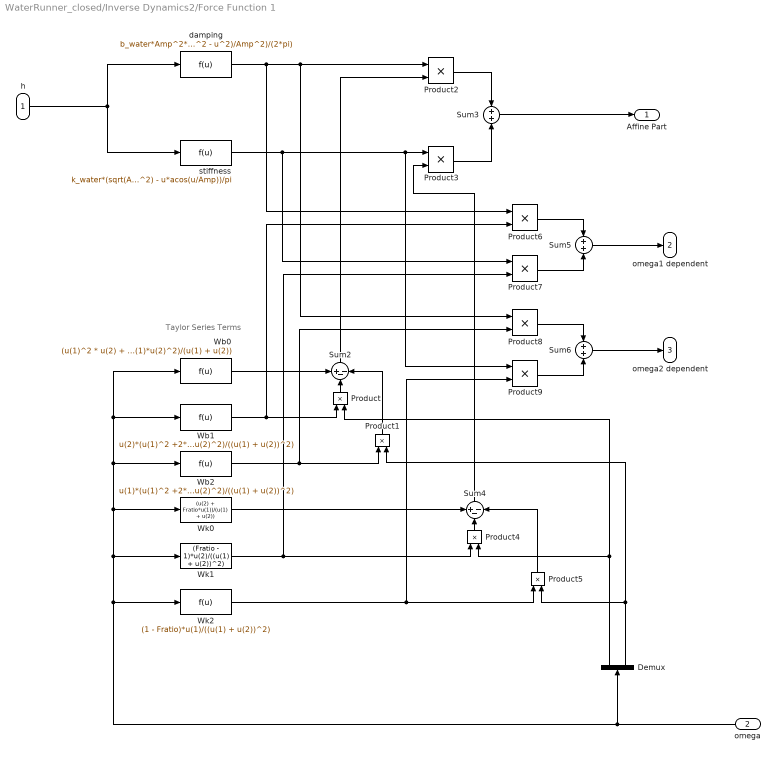
== system WaterRunner_closed/Inverse Dynamics2/Force Function 1 ==
  note: Taylor Series Terms
  h : Inport
  omega : Inport  Port=2
  Demux : Demux  Outputs=2
  Product{,1..9} (10 alike) : Product  RndMeth=Zero
  Sum2 : Sum  Inputs=+--
  Sum3 : Sum  Inputs=+|+
  Sum4 : Sum  Inputs=+--
  Sum5 : Sum  Inputs=+|+
  Sum6 : Sum  Inputs=+|+
  Wb0 : Fcn  Expr=(u(1)^2 * u(2) + Fratio*u(1)*u(2)^2)/(u(1) + u(2))
  Wb1 : Fcn  Expr=u(2)*(u(1)^2 +2*u(1)*u(2) + Fratio*u(2)^2)/((u(1) + u(2))^2)
  Wb2 : Fcn  Expr=u(1)*(u(1)^2 +2*Fratio*u(1)*u(2) + Fratio*u(2)^2)/((u(1) + u(2))^2)
  Wk0 : Fcn  Expr=(u(2) + Fratio*u(1))/(u(1) + u(2))
  Wk1 : Fcn  Expr=(Fratio - 1)*u(2)/((u(1) + u(2))^2)
  Wk2 : Fcn  Expr=(1 - Fratio)*u(1)/((u(1) + u(2))^2)
  damping : Fcn  Expr=b_water*Amp^2*(acos(u/Amp) - u*sqrt(Amp^2 - u^2)/Amp^2)/(2*pi)
  stiffness : Fcn  Expr=k_water*(sqrt(Amp^2 - u^2) - u*acos(u/Amp))/pi
  Affine Part : Outport
  omega1 dependent : Outport  Port=2
  omega2 dependent : Outport  Port=3
  wires:
  Product2/1 -> Sum3/1
  Product9/1 -> Sum6/2
  Wb1/1 -> Product6/2, Product/1
  Product4/1 -> Sum4/2
  Wb0/1 -> Sum2/1
  Product7/1 -> Sum5/2
  Wk1/1 -> Product7/2, Product4/1
  Wk0/1 -> Sum4/1
  Product6/1 -> Sum5/1
  Wb2/1 -> Product8/2, Product1/1
  Product/1 -> Sum2/2
  Sum3/1 -> Affine Part/1
  Product1/1 -> Sum2/3
  stiffness/1 -> Product7/1, Product9/1, Product3/1
  Wk2/1 -> Product5/1, Product9/2
  damping/1 -> Product6/1, Product8/1, Product2/1
  Product5/1 -> Sum4/3
  Product3/1 -> Sum3/2
  Sum5/1 -> omega1 dependent/1
  Sum4/1 -> Product3/2
  omega/1 -> Wb0/1, Wb1/1, Wb2/1, Wk0/1, Wk1/1, Wk2/1, Demux/1
  Sum2/1 -> Product2/2
  Product8/1 -> Sum6/1
  Sum6/1 -> omega2 dependent/1
  Demux/1 -> Product4/2, Product/2
  Demux/2 -> Product5/2, Product1/2
  h/1 -> stiffness/1, damping/1

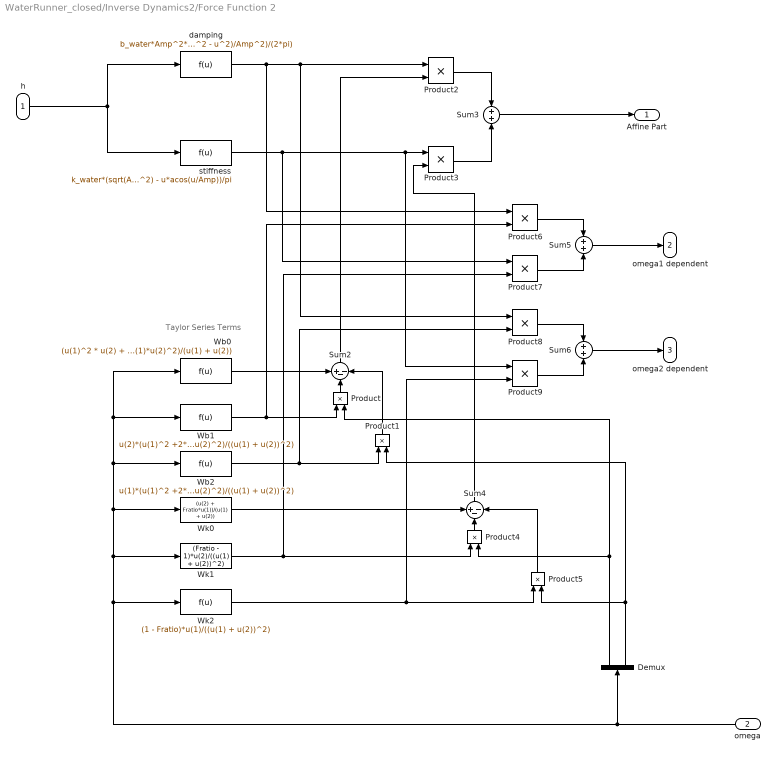
== system WaterRunner_closed/Inverse Dynamics2/Force Function 2 ==
  note: Taylor Series Terms
  h : Inport
  omega : Inport  Port=2
  Demux : Demux  Outputs=2
  Product{,1..9} (10 alike) : Product  RndMeth=Zero
  Sum2 : Sum  Inputs=+--
  Sum3 : Sum  Inputs=+|+
  Sum4 : Sum  Inputs=+--
  Sum5 : Sum  Inputs=+|+
  Sum6 : Sum  Inputs=+|+
  Wb0 : Fcn  Expr=(u(1)^2 * u(2) + Fratio*u(1)*u(2)^2)/(u(1) + u(2))
  Wb1 : Fcn  Expr=u(2)*(u(1)^2 +2*u(1)*u(2) + Fratio*u(2)^2)/((u(1) + u(2))^2)
  Wb2 : Fcn  Expr=u(1)*(u(1)^2 +2*Fratio*u(1)*u(2) + Fratio*u(2)^2)/((u(1) + u(2))^2)
  Wk0 : Fcn  Expr=(u(2) + Fratio*u(1))/(u(1) + u(2))
  Wk1 : Fcn  Expr=(Fratio - 1)*u(2)/((u(1) + u(2))^2)
  Wk2 : Fcn  Expr=(1 - Fratio)*u(1)/((u(1) + u(2))^2)
  damping : Fcn  Expr=b_water*Amp^2*(acos(u/Amp) - u*sqrt(Amp^2 - u^2)/Amp^2)/(2*pi)
  stiffness : Fcn  Expr=k_water*(sqrt(Amp^2 - u^2) - u*acos(u/Amp))/pi
  Affine Part : Outport
  omega1 dependent : Outport  Port=2
  omega2 dependent : Outport  Port=3
  wires:
  Product2/1 -> Sum3/1
  Product9/1 -> Sum6/2
  Wb1/1 -> Product6/2, Product/1
  Product4/1 -> Sum4/2
  Wb0/1 -> Sum2/1
  Product7/1 -> Sum5/2
  Wk1/1 -> Product7/2, Product4/1
  Wk0/1 -> Sum4/1
  Product6/1 -> Sum5/1
  Wb2/1 -> Product8/2, Product1/1
  Product/1 -> Sum2/2
  Sum3/1 -> Affine Part/1
  Product1/1 -> Sum2/3
  stiffness/1 -> Product7/1, Product9/1, Product3/1
  Wk2/1 -> Product5/1, Product9/2
  damping/1 -> Product6/1, Product8/1, Product2/1
  Product5/1 -> Sum4/3
  Product3/1 -> Sum3/2
  Sum5/1 -> omega1 dependent/1
  Sum4/1 -> Product3/2
  omega/1 -> Wb0/1, Wb1/1, Wb2/1, Wk0/1, Wk1/1, Wk2/1, Demux/1
  Sum2/1 -> Product2/2
  Product8/1 -> Sum6/1
  Sum6/1 -> omega2 dependent/1
  Demux/1 -> Product4/2, Product/2
  Demux/2 -> Product5/2, Product1/2
  h/1 -> stiffness/1, damping/1

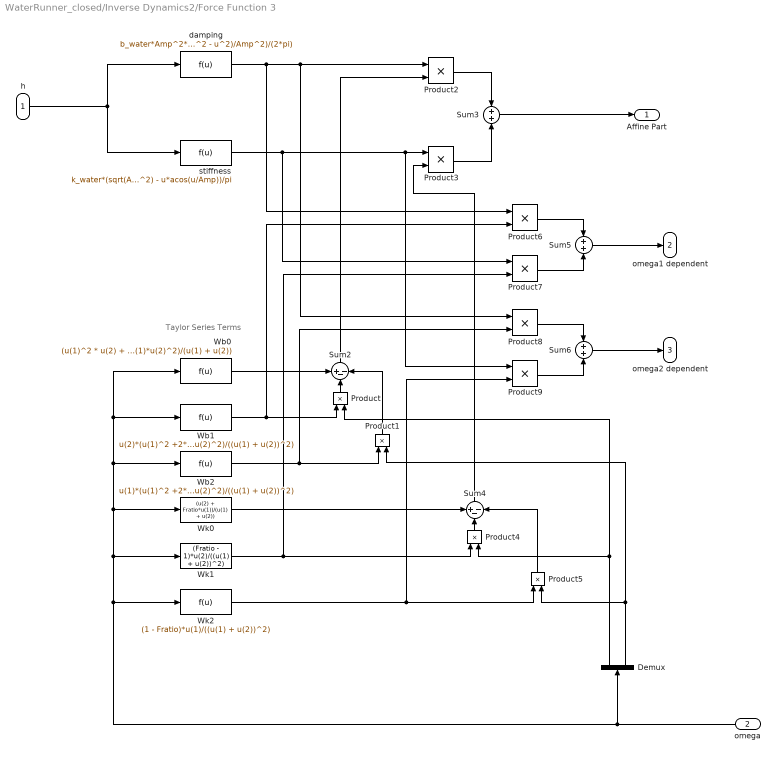
== system WaterRunner_closed/Inverse Dynamics2/Force Function 3 ==
  note: Taylor Series Terms
  h : Inport
  omega : Inport  Port=2
  Demux : Demux  Outputs=2
  Product{,1..9} (10 alike) : Product  RndMeth=Zero
  Sum2 : Sum  Inputs=+--
  Sum3 : Sum  Inputs=+|+
  Sum4 : Sum  Inputs=+--
  Sum5 : Sum  Inputs=+|+
  Sum6 : Sum  Inputs=+|+
  Wb0 : Fcn  Expr=(u(1)^2 * u(2) + Fratio*u(1)*u(2)^2)/(u(1) + u(2))
  Wb1 : Fcn  Expr=u(2)*(u(1)^2 +2*u(1)*u(2) + Fratio*u(2)^2)/((u(1) + u(2))^2)
  Wb2 : Fcn  Expr=u(1)*(u(1)^2 +2*Fratio*u(1)*u(2) + Fratio*u(2)^2)/((u(1) + u(2))^2)
  Wk0 : Fcn  Expr=(u(2) + Fratio*u(1))/(u(1) + u(2))
  Wk1 : Fcn  Expr=(Fratio - 1)*u(2)/((u(1) + u(2))^2)
  Wk2 : Fcn  Expr=(1 - Fratio)*u(1)/((u(1) + u(2))^2)
  damping : Fcn  Expr=b_water*Amp^2*(acos(u/Amp) - u*sqrt(Amp^2 - u^2)/Amp^2)/(2*pi)
  stiffness : Fcn  Expr=k_water*(sqrt(Amp^2 - u^2) - u*acos(u/Amp))/pi
  Affine Part : Outport
  omega1 dependent : Outport  Port=2
  omega2 dependent : Outport  Port=3
  wires:
  Product2/1 -> Sum3/1
  Product9/1 -> Sum6/2
  Wb1/1 -> Product6/2, Product/1
  Product4/1 -> Sum4/2
  Wb0/1 -> Sum2/1
  Product7/1 -> Sum5/2
  Wk1/1 -> Product7/2, Product4/1
  Wk0/1 -> Sum4/1
  Product6/1 -> Sum5/1
  Wb2/1 -> Product8/2, Product1/1
  Product/1 -> Sum2/2
  Sum3/1 -> Affine Part/1
  Product1/1 -> Sum2/3
  stiffness/1 -> Product7/1, Product9/1, Product3/1
  Wk2/1 -> Product5/1, Product9/2
  damping/1 -> Product6/1, Product8/1, Product2/1
  Product5/1 -> Sum4/3
  Product3/1 -> Sum3/2
  Sum5/1 -> omega1 dependent/1
  Sum4/1 -> Product3/2
  omega/1 -> Wb0/1, Wb1/1, Wb2/1, Wk0/1, Wk1/1, Wk2/1, Demux/1
  Sum2/1 -> Product2/2
  Product8/1 -> Sum6/1
  Sum6/1 -> omega2 dependent/1
  Demux/1 -> Product4/2, Product/2
  Demux/2 -> Product5/2, Product1/2
  h/1 -> stiffness/1, damping/1

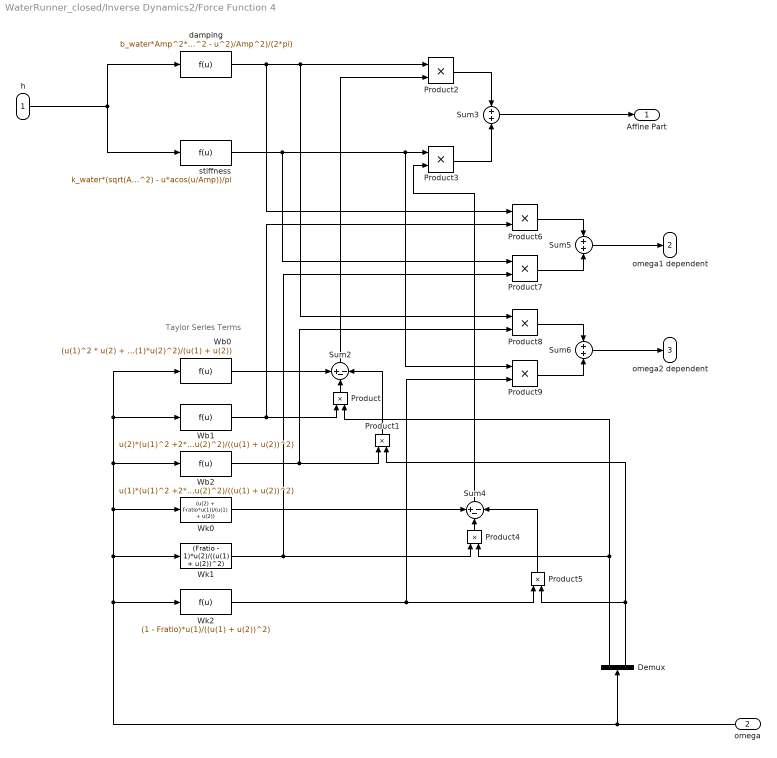
== system WaterRunner_closed/Inverse Dynamics2/Force Function 4 ==
  note: Taylor Series Terms
  h : Inport
  omega : Inport  Port=2
  Demux : Demux  Outputs=2
  Product{,1..9} (10 alike) : Product  RndMeth=Zero
  Sum2 : Sum  Inputs=+--
  Sum3 : Sum  Inputs=+|+
  Sum4 : Sum  Inputs=+--
  Sum5 : Sum  Inputs=+|+
  Sum6 : Sum  Inputs=+|+
  Wb0 : Fcn  Expr=(u(1)^2 * u(2) + Fratio*u(1)*u(2)^2)/(u(1) + u(2))
  Wb1 : Fcn  Expr=u(2)*(u(1)^2 +2*u(1)*u(2) + Fratio*u(2)^2)/((u(1) + u(2))^2)
  Wb2 : Fcn  Expr=u(1)*(u(1)^2 +2*Fratio*u(1)*u(2) + Fratio*u(2)^2)/((u(1) + u(2))^2)
  Wk0 : Fcn  Expr=(u(2) + Fratio*u(1))/(u(1) + u(2))
  Wk1 : Fcn  Expr=(Fratio - 1)*u(2)/((u(1) + u(2))^2)
  Wk2 : Fcn  Expr=(1 - Fratio)*u(1)/((u(1) + u(2))^2)
  damping : Fcn  Expr=b_water*Amp^2*(acos(u/Amp) - u*sqrt(Amp^2 - u^2)/Amp^2)/(2*pi)
  stiffness : Fcn  Expr=k_water*(sqrt(Amp^2 - u^2) - u*acos(u/Amp))/pi
  Affine Part : Outport
  omega1 dependent : Outport  Port=2
  omega2 dependent : Outport  Port=3
  wires:
  Product2/1 -> Sum3/1
  Product9/1 -> Sum6/2
  Wb1/1 -> Product6/2, Product/1
  Product4/1 -> Sum4/2
  Wb0/1 -> Sum2/1
  Product7/1 -> Sum5/2
  Wk1/1 -> Product7/2, Product4/1
  Wk0/1 -> Sum4/1
  Product6/1 -> Sum5/1
  Wb2/1 -> Product8/2, Product1/1
  Product/1 -> Sum2/2
  Sum3/1 -> Affine Part/1
  Product1/1 -> Sum2/3
  stiffness/1 -> Product7/1, Product9/1, Product3/1
  Wk2/1 -> Product5/1, Product9/2
  damping/1 -> Product6/1, Product8/1, Product2/1
  Product5/1 -> Sum4/3
  Product3/1 -> Sum3/2
  Sum5/1 -> omega1 dependent/1
  Sum4/1 -> Product3/2
  omega/1 -> Wb0/1, Wb1/1, Wb2/1, Wk0/1, Wk1/1, Wk2/1, Demux/1
  Sum2/1 -> Product2/2
  Product8/1 -> Sum6/1
  Sum6/1 -> omega2 dependent/1
  Demux/1 -> Product4/2, Product/2
  Demux/2 -> Product5/2, Product1/2
  h/1 -> stiffness/1, damping/1

== system WaterRunner_closed/Inverse Dynamics2/PID ==
  In1 : Inport
  Derivative Gain : Gain  Gain=D  Multiplication=Matrix(K*u)
  Gain : Gain  Gain=Filter_Coef
  Integral Gain : Gain  DisableCoverage=on  Gain=I  Multiplication=Matrix(K*u)
  Integrator : Integrator
  Integrator1 : Integrator
  Proportional Gain : Gain  Gain=P  Multiplication=Matrix(K*u)
  Sum : Sum  Inputs=|+-
  Sum11 : Sum  Inputs=+++
  Out1 : Outport
  wires:
  Proportional Gain/1 -> Sum11/1
  Integral Gain/1 -> Integrator/1
  Sum11/1 -> Out1/1
  Integrator/1 -> Sum11/2
  Gain/1 -> Sum11/3, Integrator1/1
  In1/1 -> Derivative Gain/1, Integral Gain/1, Proportional Gain/1
  Derivative Gain/1 -> Sum/1
  Sum/1 -> Gain/1
  Integrator1/1 -> Sum/2

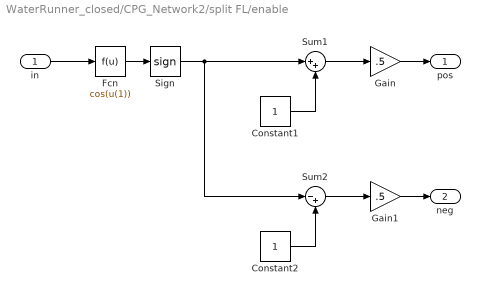
== system WaterRunner_closed/CPG_Network2/split FL/enable ==
  in : Inport
  Constant1 : Constant
  Constant2 : Constant
  Fcn : Fcn  Expr=cos(u(1))
  Gain : Gain  Gain=.5
  Gain1 : Gain  Gain=.5
  Sign : Signum
  Sum1 : Sum  Inputs=|++
  Sum2 : Sum  Inputs=|-+
  pos : Outport
  neg : Outport  Port=2
  wires:
  Fcn/1 -> Sign/1
  Constant1/1 -> Sum1/2
  Sign/1 -> Sum2/1, Sum1/1
  Gain/1 -> pos/1
  in/1 -> Fcn/1
  Sum1/1 -> Gain/1
  Constant2/1 -> Sum2/2
  Gain1/1 -> neg/1
  Sum2/1 -> Gain1/1

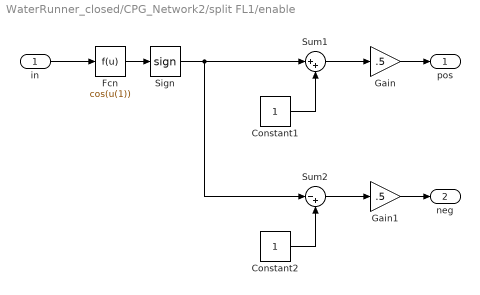
== system WaterRunner_closed/CPG_Network2/split FL1/enable ==
  in : Inport
  Constant1 : Constant
  Constant2 : Constant
  Fcn : Fcn  Expr=cos(u(1))
  Gain : Gain  Gain=.5
  Gain1 : Gain  Gain=.5
  Sign : Signum
  Sum1 : Sum  Inputs=|++
  Sum2 : Sum  Inputs=|-+
  pos : Outport
  neg : Outport  Port=2
  wires:
  Fcn/1 -> Sign/1
  Constant1/1 -> Sum1/2
  Sign/1 -> Sum2/1, Sum1/1
  Gain/1 -> pos/1
  in/1 -> Fcn/1
  Sum1/1 -> Gain/1
  Constant2/1 -> Sum2/2
  Gain1/1 -> neg/1
  Sum2/1 -> Gain1/1

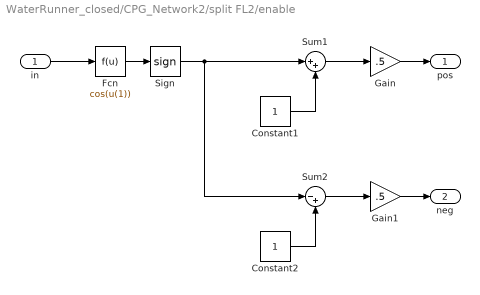
== system WaterRunner_closed/CPG_Network2/split FL2/enable ==
  in : Inport
  Constant1 : Constant
  Constant2 : Constant
  Fcn : Fcn  Expr=cos(u(1))
  Gain : Gain  Gain=.5
  Gain1 : Gain  Gain=.5
  Sign : Signum
  Sum1 : Sum  Inputs=|++
  Sum2 : Sum  Inputs=|-+
  pos : Outport
  neg : Outport  Port=2
  wires:
  Sum2/1 -> Gain1/1
  Gain1/1 -> neg/1
  Constant2/1 -> Sum2/2
  Sum1/1 -> Gain/1
  in/1 -> Fcn/1
  Gain/1 -> pos/1
  Sign/1 -> Sum1/1, Sum2/1
  Constant1/1 -> Sum1/2
  Fcn/1 -> Sign/1

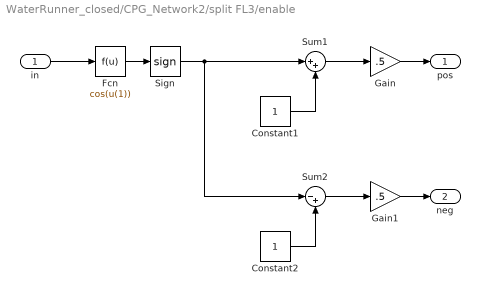
== system WaterRunner_closed/CPG_Network2/split FL3/enable ==
  in : Inport
  Constant1 : Constant
  Constant2 : Constant
  Fcn : Fcn  Expr=cos(u(1))
  Gain : Gain  Gain=.5
  Gain1 : Gain  Gain=.5
  Sign : Signum
  Sum1 : Sum  Inputs=|++
  Sum2 : Sum  Inputs=|-+
  pos : Outport
  neg : Outport  Port=2
  wires:
  Fcn/1 -> Sign/1
  Constant1/1 -> Sum1/2
  Sign/1 -> Sum2/1, Sum1/1
  Gain/1 -> pos/1
  in/1 -> Fcn/1
  Sum1/1 -> Gain/1
  Constant2/1 -> Sum2/2
  Gain1/1 -> neg/1
  Sum2/1 -> Gain1/1
